simulink model "BLAC0_velocità"  (R2025b)
settings: Solver=FixedStepAuto  StartTime=0.0  StopTime=0.1  FixedStep=1e-4  RelTol=1e-3
values from neighbouring files (symbols this model uses):
  B = 3.8e-005    (= 3.8e-05)    [Dati0_1.m]
  Crn = 0.6    [Dati0_1.m]
  J = 0.0000251    (= 2.51e-05)    [Dati0_1.m]
  Kc = ms*np*lambdaf/2    (= 0.27)    [Dati0_1.m]
  Lsd = 0.005/2    (= 0.0025)    [Dati0_1.m]
  Lsq = Lsd    (= 0.0025)    [Dati0_1.m]
  np = 2    [Dati0_1.m]
  PSIPM = lambdaf    (= 0.09)    [Dati0_1.m]
  Rs = 3.1/2    (= 1.55)    [Dati0_1.m]
  wrr = 1256.6    [Dati0_1.m]
settings Model: Creator=Nicolas  LastModifiedBy=Steph
settings DataIOCC: ReturnWorkspaceOutputs=off

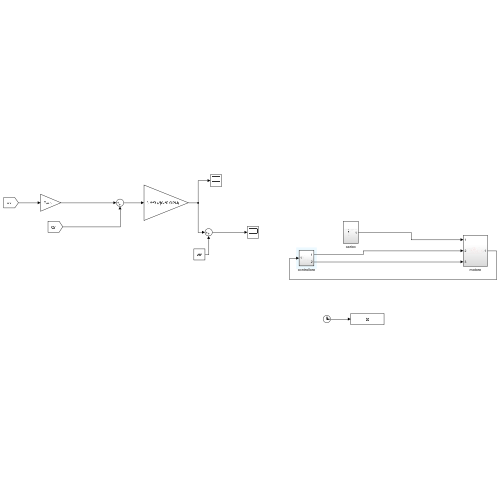
[thumbnail: Simulink's stored preview of the top-level diagram]
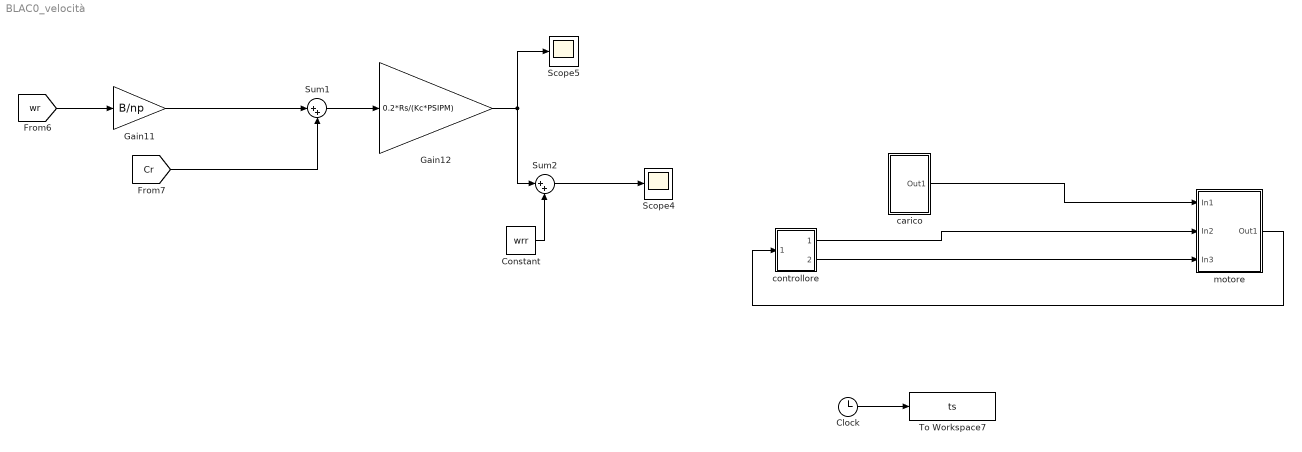
== system BLAC0_velocità ==
  Clock : Clock
  Constant : Constant  Value=wrr
  Gain11 : Gain  Gain=B/np
  Gain12 : Gain  Gain=0.2*Rs/(Kc*PSIPM)
  Scope4 : Scope
      settings: ActiveDisplayYMinimum=1239.82875  ActiveDisplayYMaximum=1266.36927
  Scope5 : Scope
      settings: ActiveDisplayYMinimum=7.17571  ActiveDisplayYMaximum=8.48624  DataLoggingVariableName=ScopeData2
  Sum1 : Sum  Inputs=|++
  Sum2 : Sum  Inputs=|++
  To Workspace7 : ToWorkspace  VariableName=ts  SaveFormat=Timeseries  SampleTime=-1
  carico : Subsystem
  controllore : Subsystem
  motore : Subsystem
  wires:
  Clock/1 -> To Workspace7/1
  [wr] -> Gain11/1
  Gain11/1 -> Sum1/1
  [Cr] -> Sum1/2
  Sum1/1 -> Gain12/1
  Gain12/1 -> Sum2/1, Scope5/1
  Constant/1 -> Sum2/2
  Sum2/1 -> Scope4/1
  carico/1(Out1) -> motore/1(In1)
  controllore/1(Out1) -> motore/2(In2)
  controllore/2(Out2) -> motore/3(In3)
  motore/1(Out1) -> controllore/1(In2)

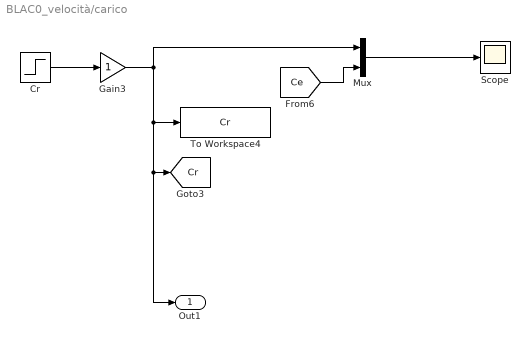
== system BLAC0_velocità/carico ==
  Cr : Step  Time=0.05  After=Crn  SampleTime=0
  Gain3 : Gain
  Mux : Mux  Inputs=2
  Scope : Scope
      settings: ActiveDisplayYMinimum=-4.0916456084062247  ActiveDisplayYMaximum=10.229860426392403
  To Workspace4 : ToWorkspace  VariableName=Cr  SaveFormat=Timeseries  SampleTime=-1
  Out1 : Outport
  tag scope: Cr=global
  wires:
  Cr/1 -> Gain3/1
  Mux/1 -> Scope/1
  [Ce] -> Mux/2
  Gain3/1 -> Out1/1, [Cr], To Workspace4/1, Mux/1

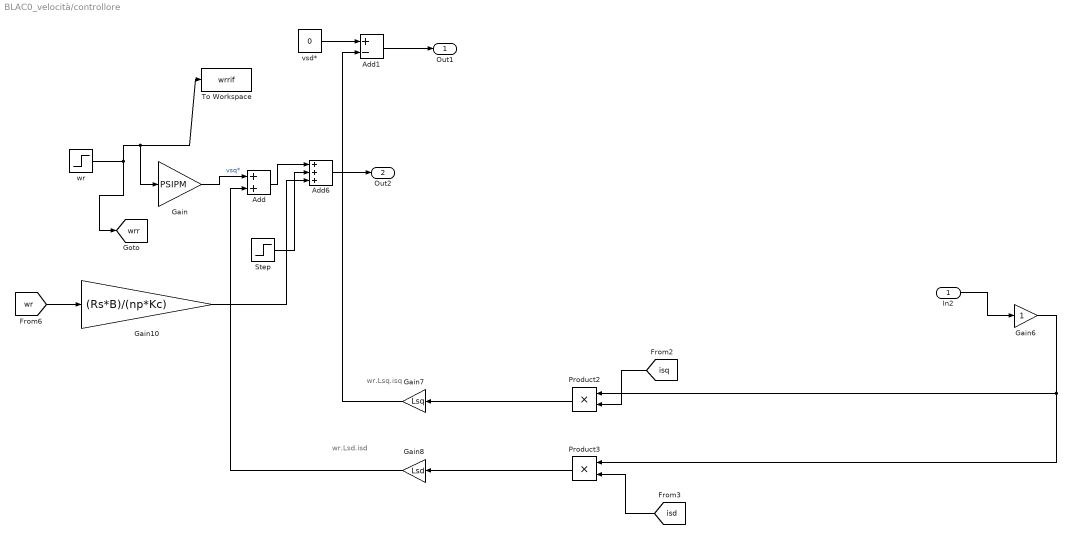
== system BLAC0_velocità/controllore ==
  note: wr.Lsd.isd
  note: wr.Lsq.isq
  In2 : Inport
  Add : Sum
  Add1 : Sum  Inputs=+-
  Add6 : Sum  Inputs=+++
  Gain : Gain  Gain=PSIPM
  Gain10 : Gain  Gain=(Rs*B)/(np*Kc)
  Gain6 : Gain
  Gain7 : Gain  Gain=Lsq
  Gain8 : Gain  Gain=Lsd
  Product2 : Product
  Product3 : Product
  Step : Step  Time=0.05  After=Rs*Crn/Kc  SampleTime=0
  To Workspace : ToWorkspace  VariableName=wrrif  SaveFormat=Timeseries  SampleTime=-1
  vsd* : Constant  Value=0
  wr : Step  Time=0  After=1256.6  SampleTime=0
  Out1 : Outport
  Out2 : Outport  Port=2
  tag scope: wrr=global
  wires:
  Gain7/1 -> Add1/2
  vsd*/1 -> Add1/1
  [isd] -> Product3/2
  Product3/1 -> Gain8/1
  Add/1 -> Add6/1
  wr/1 -> [wrr], To Workspace/1, Gain/1
  Gain/1 -> Add/1  "vsq*"
  [isq] -> Product2/2
  In2/1 -> Gain6/1
  Product2/1 -> Gain7/1
  Gain6/1 -> Product3/1, Product2/1
  [wr] -> Gain10/1
  Gain8/1 -> Add/2
  Add1/1 -> Out1/1
  Add6/1 -> Out2/1
  Step/1 -> Add6/2
  Gain10/1 -> Add6/3

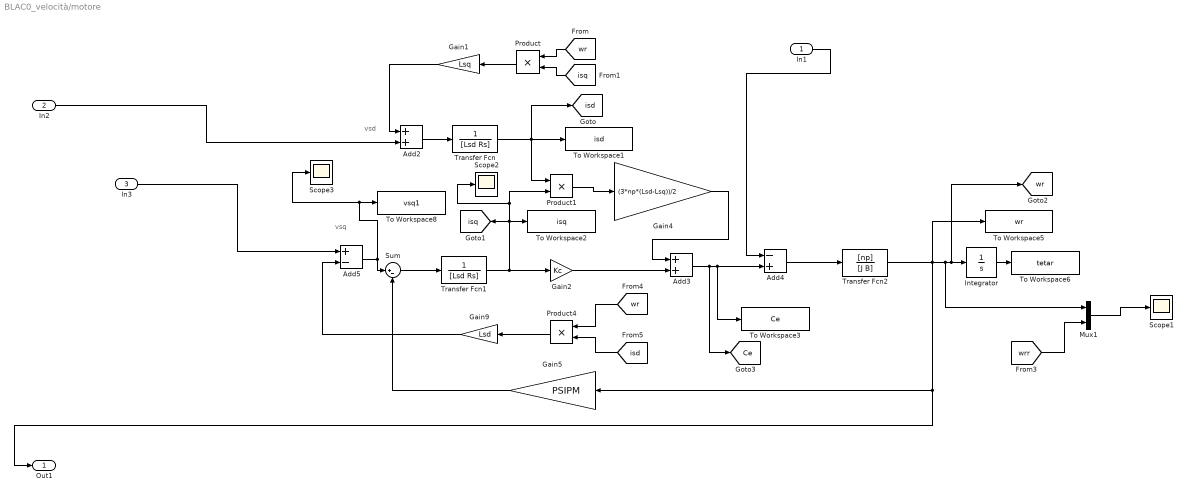
== system BLAC0_velocità/motore ==
  note: vsd
  note: vsq
  In1 : Inport
  In2 : Inport  Port=2
  In3 : Inport  Port=3
  Add2 : Sum
  Add3 : Sum
  Add4 : Sum  Inputs=-+
  Add5 : Sum  Inputs=+-
  Gain1 : Gain  Gain=Lsq
  Gain2 : Gain  Gain=Kc
  Gain4 : Gain  Gain=(3*np*(Lsd-Lsq))/2
  Gain5 : Gain  Gain=PSIPM
  Gain9 : Gain  Gain=Lsd
  Integrator : Integrator
  Mux1 : Mux  Inputs=2
  Product : Product
  Product1 : Product
  Product4 : Product
  Scope1 : Scope
      settings: ActiveDisplayYMinimum=-205.05890249206215  ActiveDisplayYMaximum=1845.53012242856
  Scope2 : Scope
      settings: ActiveDisplayYMinimum=-15.15118  ActiveDisplayYMaximum=37.90229
  Scope3 : Scope
      settings: ActiveDisplayYMinimum=112.64617  ActiveDisplayYMaximum=117.12449  DataLoggingVariableName=ScopeData2
  Sum : Sum  Inputs=|+-
  To Workspace1 : ToWorkspace  VariableName=isd  SaveFormat=Timeseries  SampleTime=-1
  To Workspace2 : ToWorkspace  VariableName=isq  SaveFormat=Timeseries  SampleTime=-1
  To Workspace3 : ToWorkspace  VariableName=Ce  SaveFormat=Timeseries  SampleTime=-1
  To Workspace5 : ToWorkspace  VariableName=wr  SaveFormat=Timeseries  SampleTime=-1
  To Workspace6 : ToWorkspace  VariableName=tetar  SaveFormat=Timeseries  SampleTime=-1
  To Workspace8 : ToWorkspace  VariableName=vsq1  SaveFormat=Timeseries  SampleTime=-1
  Transfer Fcn : TransferFcn  Denominator=[Lsd Rs]
  Transfer Fcn1 : TransferFcn  Denominator=[Lsd Rs]
  Transfer Fcn2 : TransferFcn  Numerator=[np]  Denominator=[J B]
  Out1 : Outport
  tag scope: Ce=global, isd=global, isq=global, wr=global
  wires:
  Transfer Fcn/1 -> [isd], To Workspace1/1, Product1/1
  Mux1/1 -> Scope1/1
  Transfer Fcn2/1 -> Out1/1, Gain5/1, To Workspace5/1, Mux1/1, [wr], Integrator/1
  Add5/1 -> To Workspace8/1, Scope3/1, Sum/1
  Product1/1 -> Gain4/1
  Gain9/1 -> Add5/2
  Integrator/1 -> To Workspace6/1
  Transfer Fcn1/1 -> Scope2/1, Product1/2, [isq], To Workspace2/1, Gain2/1
  In2/1 -> Add2/2
  Add2/1 -> Transfer Fcn/1
  Product/1 -> Gain1/1
  Add3/1 -> [Ce], Add4/2, To Workspace3/1
  Gain5/1 -> Sum/2
  Gain4/1 -> Add3/1
  In3/1 -> Add5/1
  [wr] -> Product4/1
  [wr] -> Product/1
  Product4/1 -> Gain9/1
  Sum/1 -> Transfer Fcn1/1
  [isq] -> Product/2
  Gain2/1 -> Add3/2
  Add4/1 -> Transfer Fcn2/1
  [isd] -> Product4/2
  [wrr] -> Mux1/2
  Gain1/1 -> Add2/1
  In1/1 -> Add4/1
